simulink model "MLC_PreEval"  (Simulink 10.1)
settings: Solver=ode4  StartTime=0.0  StopTime=Parameter.Time.TMax  FixedStep=Parameter.Time.dt  MaxStep=10*Parameter.Time.dt  MinStep=Parameter.Time.dt  RelTol=1e-3  EnableMultiTasking=on
undefined symbols (not defined in the file or in its folder): Parameter, x2_t0
libraries: simulink x1
settings Model: Creator=Phoenix_Shao  LastModifiedBy=jveli
settings SolverCC: InitialStep=4*Parameter.Time.dt  MaxConsecutiveMinStep=10
settings DataIOCC: MaxDataPoints=1000000  SaveFormat=Dataset  SignalLogging=off  DSMLogging=off
settings OptimizationCC: ExpressionDepthLimit=2147483647  InitFltsAndDblsToZero=on  EfficientMapNaN2IntZero=off
settings DebuggingCC: SaveWithParameterizedLinksMsg=none  SignalResolutionControl=TryResolveAllWithWarning  SolverPrmCheckMsg=warning  MultiTaskDSMMsg=warning  MultiTaskCondExecSysMsg=none  FcnCallInpInsideContextMsg=warning  AllowSymbolicDim=off  StateNameClashWarn=warning
settings HardwareCC: TargetBitPerPointer=64  TargetBitPerSizeT=64  TargetBitPerPtrDiffT=64  TargetLongLongMode=on  TargetIntDivRoundTo=Zero  TargetEndianess=LittleEndian  TargetWordSize=64  TargetHWDeviceType=MATLAB Host  ProdEqTarget=off
settings ModelReferenceCC: ModelDependencies=|
  | MAP_x64.dll
  | OpenFAST-Simulink_x64.dll
  | FAST_SFunc.mexw64
settings SFSimCC: SimParseCustomCode=off
settings RTWCC: SystemTargetFile=accel.tlc  TemplateMakefile=accel_default_tmf  RTWVerbose=off
settings CodeAppCC: MaxIdLength=128
settings STFCustomTargetCC: MATLABClassNameForMDSCustomization=Simulink.SoftwareTarget.TargetSpecificTriggerConfigurationBase  SystemTargetFile=accel.tlc

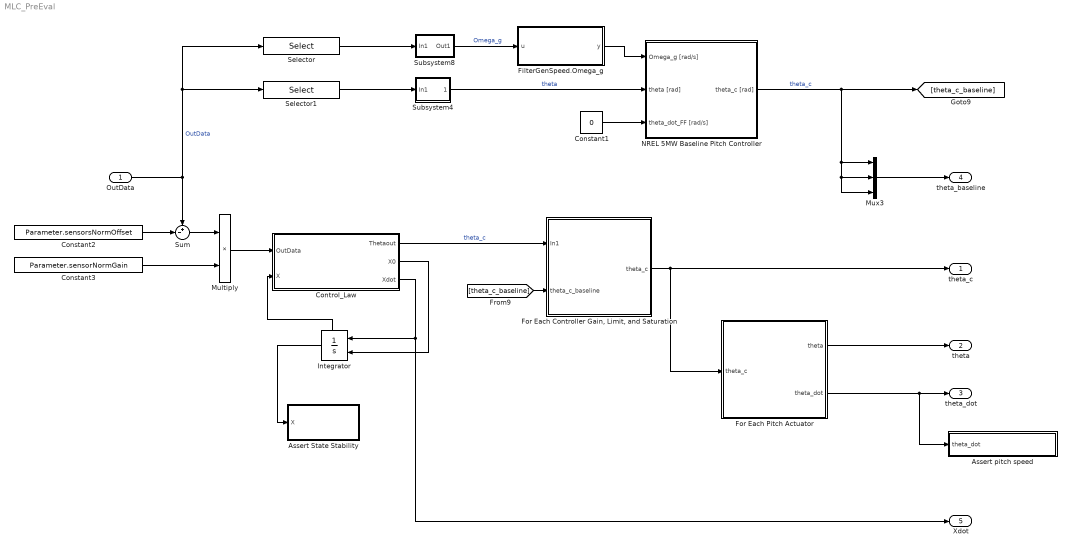
== system MLC_PreEval ==
  OutData : Inport  PortDimensions=Parameter.MLC.totNSensors
  Assert State Stability : Subsystem
  Assert pitch speed : Subsystem
  Constant1 : Constant  Value=0
  Constant2 : Constant  Value=Parameter.sensorsNormOffset
  Constant3 : Constant  Value=Parameter.sensorNormGain
  Control_Law : MATLAB Function  TreatAsAtomicUnit=on
  FilterGenSpeed.Omega_g : Subsystem
  For Each Pitch Actuator : Subsystem  TreatAsAtomicUnit=on
  "For Each Controller Gain, Limit, and Saturation" : Subsystem  TreatAsAtomicUnit=on
  Integrator : Integrator  InitialConditionSource=external  ShowStatePort=on
  Multiply : Product
  Mux3 : Mux  Inputs=3
  NREL 5MW Baseline Pitch Controller : Subsystem
  Selector : Selector  InputPortWidth=Parameter.outListLen  IndexOptions=Index vector (dialog)  Indices=Parameter.outListIdx.GenSpeed  OutputSizes=1
  Selector1 : Selector  InputPortWidth=Parameter.outListLen  IndexOptions=Index vector (dialog)  Indices=Parameter.outListIdx.BldPitch1  OutputSizes=1
  Subsystem4 : Subsystem
      mask Display: disp('deg2rad')
  Subsystem8 : Subsystem
      mask Display: disp('rpm2rad/s')
  Sum : Sum  Inputs=+-|
  "theta_c " : Outport  SignalName=theta_c  VectorParamsAs1DForOutWhenUnconnected=off
  theta : Outport  Port=2  SignalName=theta  VectorParamsAs1DForOutWhenUnconnected=off
  theta_dot : Outport  Port=3  SignalName=theta_dot  VectorParamsAs1DForOutWhenUnconnected=off
  theta_baseline : Outport  Port=4  SignalName=theta_baseline  VectorParamsAs1DForOutWhenUnconnected=off
  Xdot : Outport  Port=5  SignalName=Xdot  VectorParamsAs1DForOutWhenUnconnected=off
  wires:
  "For Each Controller Gain, Limit, and Saturation"/1(theta_c) -> For Each Pitch Actuator/1(theta_c), "theta_c "/1
  OutData/1 -> Selector1/1, Selector/1, Sum/1  "OutData"
  For Each Pitch Actuator/1(theta) -> theta/1
  For Each Pitch Actuator/2(theta_dot) -> Assert pitch speed/1(theta_dot), theta_dot/1
  FilterGenSpeed.Omega_g/1(y) -> NREL 5MW Baseline Pitch Controller/1(Omega_g [rad/s])
  Constant1/1 -> NREL 5MW Baseline Pitch Controller/3(theta_dot_FF [rad/s])
  Subsystem8/1(Out1) -> FilterGenSpeed.Omega_g/1(u)  "Omega_g"
  Selector/1 -> Subsystem8/1(In1)
  Subsystem4/1(Out1) -> NREL 5MW Baseline Pitch Controller/2(theta [rad])  "theta"
  Selector1/1 -> Subsystem4/1(In1)
  NREL 5MW Baseline Pitch Controller/1(theta_c [rad]) -> Mux3/1, Mux3/2, Mux3/3, [theta_c_baseline]  "theta_c"
  Constant2/1 -> Sum/2
  Sum/1 -> Multiply/1
  Constant3/1 -> Multiply/2
  Mux3/1 -> theta_baseline/1
  [theta_c_baseline] -> "For Each Controller Gain, Limit, and Saturation"/2(theta_c_baseline)
  Integrator/1 -> Assert State Stability/1(X)
  Control_Law/1(Thetaout) -> "For Each Controller Gain, Limit, and Saturation"/1(In1)  "theta_c"
  Control_Law/2(X0) -> Integrator/2
  Control_Law/3(Xdot) -> Xdot/1, Integrator/1
  Multiply/1 -> Control_Law/1(OutData)
  Integrator/State -> Control_Law/2(X)

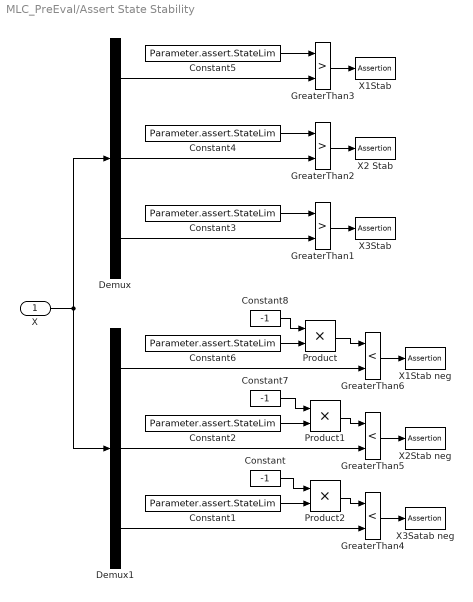
== system MLC_PreEval/Assert State Stability ==
  X : Inport
  Constant : Constant  Value=-1
  Constant{1..6} (6 alike) : Constant  Value=Parameter.assert.StateLim
  Constant7 : Constant  Value=-1
  Constant8 : Constant  Value=-1
  Demux : Demux  Outputs=3
  Demux1 : Demux  Outputs=3
  GreaterThan1 : RelationalOperator  Operator=>  OutDataTypeStr=boolean  RndMeth=Simplest
  GreaterThan2 : RelationalOperator  Operator=>  OutDataTypeStr=boolean  RndMeth=Simplest
  GreaterThan3 : RelationalOperator  Operator=>  OutDataTypeStr=boolean  RndMeth=Simplest
  GreaterThan4 : RelationalOperator  Operator=<  OutDataTypeStr=boolean  RndMeth=Simplest
  GreaterThan5 : RelationalOperator  Operator=<  OutDataTypeStr=boolean  RndMeth=Simplest
  GreaterThan6 : RelationalOperator  Operator=<  OutDataTypeStr=boolean  RndMeth=Simplest
  Product : Product
  Product1 : Product
  Product2 : Product
  X1Stab : Assertion
  X1Stab neg : Assertion
  X2 Stab : Assertion
  X2Stab neg : Assertion
  X3Satab neg : Assertion
  X3Stab : Assertion
  wires:
  Constant5/1 -> GreaterThan3/1
  GreaterThan1/1 -> X3Stab/1
  Constant3/1 -> GreaterThan1/1
  Constant4/1 -> GreaterThan2/1
  GreaterThan3/1 -> X1Stab/1
  GreaterThan2/1 -> X2 Stab/1
  X/1 -> Demux/1, Demux1/1
  Demux/2 -> GreaterThan2/2
  Demux/3 -> GreaterThan1/2
  GreaterThan6/1 -> X1Stab neg/1
  Demux/1 -> GreaterThan3/2
  GreaterThan4/1 -> X3Satab neg/1
  Constant2/1 -> Product1/2
  Constant6/1 -> Product/2
  Constant1/1 -> Product2/2
  GreaterThan5/1 -> X2Stab neg/1
  Product/1 -> GreaterThan6/1
  Product1/1 -> GreaterThan5/1
  Product2/1 -> GreaterThan4/1
  Constant/1 -> Product2/1
  Constant7/1 -> Product1/1
  Constant8/1 -> Product/1
  Demux1/2 -> GreaterThan5/2
  Demux1/1 -> GreaterThan6/2
  Demux1/3 -> GreaterThan4/2

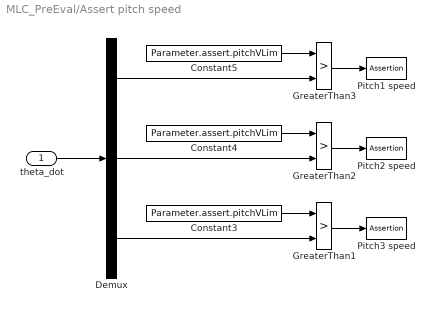
== system MLC_PreEval/Assert pitch speed ==
  theta_dot : Inport
  Constant3 : Constant  Value=Parameter.assert.pitchVLim
  Constant4 : Constant  Value=Parameter.assert.pitchVLim
  Constant5 : Constant  Value=Parameter.assert.pitchVLim
  Demux : Demux  Outputs=3
  GreaterThan1 : RelationalOperator  Operator=>  OutDataTypeStr=boolean  RndMeth=Simplest
  GreaterThan2 : RelationalOperator  Operator=>  OutDataTypeStr=boolean  RndMeth=Simplest
  GreaterThan3 : RelationalOperator  Operator=>  OutDataTypeStr=boolean  RndMeth=Simplest
  Pitch1 speed : Assertion
  Pitch2 speed : Assertion
  Pitch3 speed : Assertion
  wires:
  Constant5/1 -> GreaterThan3/1
  GreaterThan1/1 -> Pitch3 speed/1
  Constant3/1 -> GreaterThan1/1
  Constant4/1 -> GreaterThan2/1
  GreaterThan3/1 -> Pitch1 speed/1
  GreaterThan2/1 -> Pitch2 speed/1
  theta_dot/1 -> Demux/1
  Demux/1 -> GreaterThan3/2
  Demux/2 -> GreaterThan2/2
  Demux/3 -> GreaterThan1/2

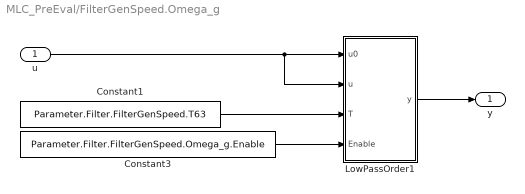
== system MLC_PreEval/FilterGenSpeed.Omega_g ==
  u : Inport
  Constant1 : Constant  Value=Parameter.Filter.FilterGenSpeed.T63
  Constant3 : Constant  Value=Parameter.Filter.FilterGenSpeed.Omega_g.Enable
  LowPassOrder1 : Subsystem
  y : Outport  VectorParamsAs1DForOutWhenUnconnected=off
  wires:
  LowPassOrder1/1(y) -> y/1
  u/1 -> LowPassOrder1/2(u), LowPassOrder1/1(u0)
  Constant3/1 -> LowPassOrder1/4(Enable)
  Constant1/1 -> LowPassOrder1/3(T)

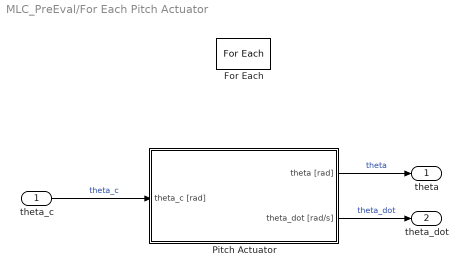
== system MLC_PreEval/For Each Pitch Actuator ==
  theta_c : Inport  Partition=on  PartitionDimension=1  PartitionWidth=1  PartitionOffset=0
  For Each : ForEach  DisableCoverage=on
  Pitch Actuator : Subsystem  AncestorBlock=Library/Models/Pitch Actuator
  theta : Outport  ConcatenationDimension=1  VectorParamsAs1DForOutWhenUnconnected=off
  theta_dot : Outport  Port=2  ConcatenationDimension=1  VectorParamsAs1DForOutWhenUnconnected=off
  wires:
  theta_c/1 -> Pitch Actuator/1(theta_c [rad])  "theta_c"
  Pitch Actuator/1(theta [rad]) -> theta/1  "theta"
  Pitch Actuator/2(theta_dot [rad/s]) -> theta_dot/1  "theta_dot"

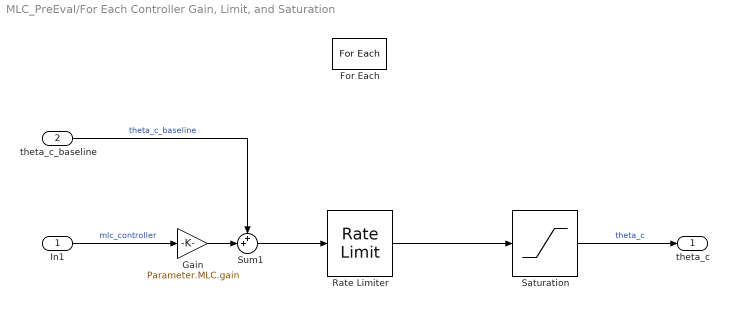
== system MLC_PreEval/For Each Controller Gain, Limit, and Saturation ==
  In1 : Inport  Partition=on  PartitionDimension=1  PartitionWidth=1  PartitionOffset=0
  theta_c_baseline : Inport  Port=2
  For Each : ForEach  DisableCoverage=on
  Gain : Gain  Gain=Parameter.MLC.gain
      settings: AttributesFormatString=%<Gain>
  Rate Limiter : RateLimiter  RisingSlewLimit=deg2rad(Parameter.assert.pitchVLim)  FallingSlewLimit=-deg2rad(Parameter.assert.pitchVLim)  SampleTimeMode=inherited
      settings: AttributesFormatString=|
      | %<RisingSlewLimit>
      | %<FallingSlewLimit>
  Saturation : Saturate  UpperLimit=Parameter.CPC.theta_max  LowerLimit=Parameter.CPC.theta_min
      settings: AttributesFormatString=|
      | %<UpperLimit>
      | %<LowerLimit>
  Sum1 : Sum  Inputs=++|
  theta_c : Outport  ConcatenationDimension=1  VectorParamsAs1DForOutWhenUnconnected=off
  wires:
  Sum1/1 -> Rate Limiter/1
  Saturation/1 -> theta_c/1  "theta_c"
  Gain/1 -> Sum1/2
  theta_c_baseline/1 -> Sum1/1  "theta_c_baseline"
  Rate Limiter/1 -> Saturation/1
  In1/1 -> Gain/1  "mlc_controller"

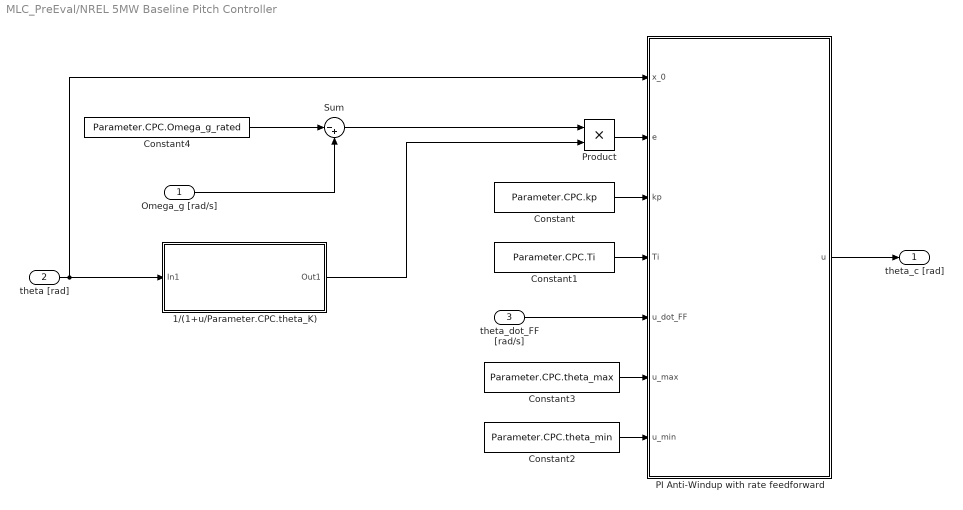
== system MLC_PreEval/NREL 5MW Baseline Pitch Controller ==
  Omega_g [rad/s] : Inport
  theta [rad] : Inport  Port=2
  theta_dot_FF [rad/s] : Inport  Port=3
  1/(1+u/Parameter.CPC.theta_K) : Subsystem
  Constant : Constant  Value=Parameter.CPC.kp
  Constant1 : Constant  Value=Parameter.CPC.Ti
  Constant2 : Constant  Value=Parameter.CPC.theta_min
  Constant3 : Constant  Value=Parameter.CPC.theta_max
  Constant4 : Constant  Value=Parameter.CPC.Omega_g_rated
  PI Anti-Windup with rate feedforward : Subsystem
  Product : Product  RndMeth=Zero
  Sum : Sum  Inputs=|-+
  theta_c [rad] : Outport  VectorParamsAs1DForOutWhenUnconnected=off
  wires:
  Constant4/1 -> Sum/1
  theta [rad]/1 -> 1/(1+u/Parameter.CPC.theta_K)/1(In1), PI Anti-Windup with rate feedforward/1(x_0)
  Omega_g [rad/s]/1 -> Sum/2
  1/(1+u/Parameter.CPC.theta_K)/1(Out1) -> Product/2
  Sum/1 -> Product/1
  Product/1 -> PI Anti-Windup with rate feedforward/2(e)
  theta_dot_FF [rad/s]/1 -> PI Anti-Windup with rate feedforward/5(u_dot_FF)
  PI Anti-Windup with rate feedforward/1(u) -> theta_c [rad]/1
  Constant/1 -> PI Anti-Windup with rate feedforward/3(kp)
  Constant1/1 -> PI Anti-Windup with rate feedforward/4(Ti)
  Constant2/1 -> PI Anti-Windup with rate feedforward/7(u_min)
  Constant3/1 -> PI Anti-Windup with rate feedforward/6(u_max)

== system MLC_PreEval/Subsystem4 ==
  In1 : Inport
  deg in rad : Gain  Gain=2*pi/360  SaturateOnIntegerOverflow=on  OutDataTypeStr=Inherit: Same as input  ParamDataTypeStr=Inherit: Same as input
  Out1 : Outport  VectorParamsAs1DForOutWhenUnconnected=off
  wires:
  In1/1 -> deg in rad/1
  deg in rad/1 -> Out1/1

== system MLC_PreEval/Subsystem8 ==
  In1 : Inport
  rpm in rad/s : Gain  Gain=2*pi/60  SaturateOnIntegerOverflow=on  OutDataTypeStr=Inherit: Same as input  ParamDataTypeStr=Inherit: Same as input
  Out1 : Outport  VectorParamsAs1DForOutWhenUnconnected=off
  wires:
  rpm in rad/s/1 -> Out1/1
  In1/1 -> rpm in rad/s/1

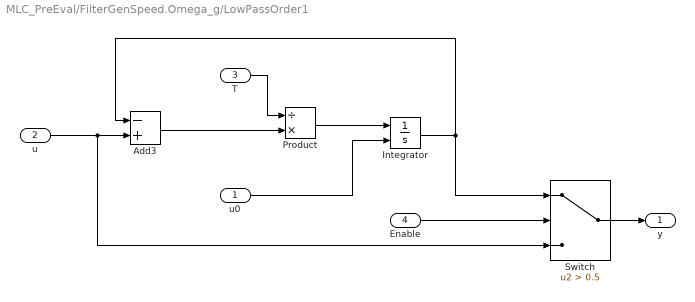
== system MLC_PreEval/FilterGenSpeed.Omega_g/LowPassOrder1 ==
  u0 : Inport
  u : Inport  Port=2
  T : Inport  Port=3
  Enable : Inport  Port=4
  Add3 : Sum  Inputs=-+
  Integrator : Integrator  InitialConditionSource=external
  Product : Product  Inputs=/*  RndMeth=Zero
  Switch : Switch  Criteria=u2 > Threshold  Threshold=0.5
  y : Outport  VectorParamsAs1DForOutWhenUnconnected=off
  wires:
  u0/1 -> Integrator/2
  Switch/1 -> y/1
  Enable/1 -> Switch/2
  u/1 -> Add3/2, Switch/3
  T/1 -> Product/1
  Integrator/1 -> Add3/1, Switch/1
  Product/1 -> Integrator/1
  Add3/1 -> Product/2

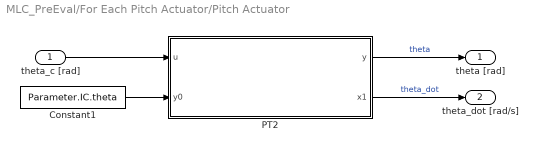
== system MLC_PreEval/For Each Pitch Actuator/Pitch Actuator ==
  theta_c [rad] : Inport
  Constant1 : Constant  Value=Parameter.IC.theta
  PT2 : Subsystem  mask{omega=Parameter.PitchActuator.omega, xi=Parameter.PitchActuator.xi, x1_max=Parameter.PitchActuator.theta_dot_max, x1_min=-Parameter.PitchActuator.theta_dot_max, x2_max=Parameter.PitchActuator.theta_max, x2_min=Parameter.PitchActuator.theta_min}
      mask prompts: omega "undamped natural frequency [rad/s]"; xi "damping factor [-]"; x1_max "Upper bound x1"; x1_min "Lower bound x1"; x2_max "Upper bound x2"; x2_min "Lower bound x2"
      mask Display:
      | disp(['omega = ',num2str(omega),'\n'...
      |     ,'xi = ',num2str(xi)])
      | port_label('output',1,'y')
      | port_label('output',2,'x1')
      | port_label('input',2,'y0')
      | port_label('input',1,'u')
  theta [rad] : Outport  VectorParamsAs1DForOutWhenUnconnected=off
  theta_dot [rad/s] : Outport  Port=2  VectorParamsAs1DForOutWhenUnconnected=off
  wires:
  Constant1/1 -> PT2/2(y0)
  theta_c [rad]/1 -> PT2/1(u)
  PT2/1(y) -> theta [rad]/1  "theta"
  PT2/2(x1) -> theta_dot [rad/s]/1  "theta_dot"

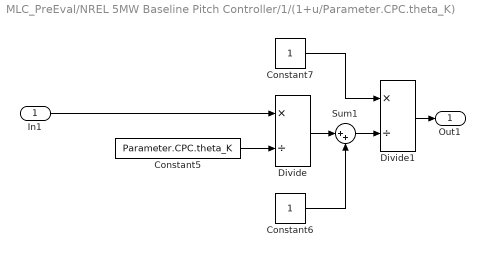
== system MLC_PreEval/NREL 5MW Baseline Pitch Controller/1/(1+u/Parameter.CPC.theta_K) ==
  In1 : Inport
  Constant5 : Constant  Value=Parameter.CPC.theta_K
  Constant6 : Constant
  Constant7 : Constant
  Divide : Product  Inputs=*/
  Divide1 : Product  Inputs=*/
  Sum1 : Sum  Inputs=|++
  Out1 : Outport  VectorParamsAs1DForOutWhenUnconnected=off
  wires:
  Sum1/1 -> Divide1/2
  Divide/1 -> Sum1/1
  In1/1 -> Divide/1
  Divide1/1 -> Out1/1
  Constant7/1 -> Divide1/1
  Constant5/1 -> Divide/2
  Constant6/1 -> Sum1/2

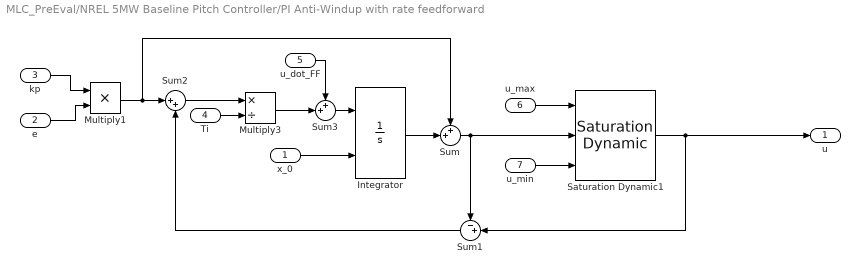
== system MLC_PreEval/NREL 5MW Baseline Pitch Controller/PI Anti-Windup with rate feedforward ==
  x_0 : Inport
  e : Inport  Port=2
  kp : Inport  Port=3
  Ti : Inport  Port=4
  u_dot_FF : Inport  Port=5
  u_max : Inport  Port=6
  u_min : Inport  Port=7
  Integrator : Integrator  InitialConditionSource=external
  Multiply1 : Product  Inputs=**
  Multiply3 : Product  Inputs=*/
  Saturation Dynamic1 : simulink/Discontinuities/Saturation Dynamic  OutMin=[]  OutMax=[]  OutDataTypeStr=Inherit: Same as second input  OutDataType=fixdt(1, 16)  OutScaling=2^-10  DoSatur=off
  Sum : Sum  Inputs=++|
  Sum1 : Sum  Inputs=-+|
  Sum2 : Sum  Inputs=|++
  Sum3 : Sum  Inputs=++|
  u : Outport  VectorParamsAs1DForOutWhenUnconnected=off
  wires:
  Saturation Dynamic1/1 -> u/1, Sum1/2
  Integrator/1 -> Sum/2
  kp/1 -> Multiply1/1
  e/1 -> Multiply1/2
  Ti/1 -> Multiply3/2
  Multiply1/1 -> Sum/1, Sum2/1
  Sum2/1 -> Multiply3/1
  x_0/1 -> Integrator/2
  Multiply3/1 -> Sum3/2
  Sum3/1 -> Integrator/1
  u_dot_FF/1 -> Sum3/1
  u_min/1 -> Saturation Dynamic1/3
  Sum/1 -> Saturation Dynamic1/2, Sum1/1
  u_max/1 -> Saturation Dynamic1/1
  Sum1/1 -> Sum2/2

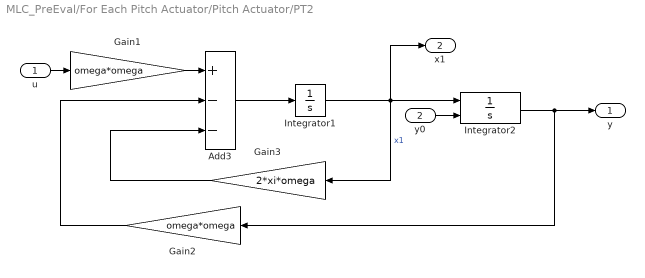
== system MLC_PreEval/For Each Pitch Actuator/Pitch Actuator/PT2 ==
  u : Inport
  y0 : Inport  Port=2
  Add3 : Sum  Inputs=+--
  Gain1 : Gain  Gain=omega*omega  SaturateOnIntegerOverflow=on  OutDataTypeStr=Inherit: Same as input  ParamDataTypeStr=Inherit: Same as input
  Gain2 : Gain  Gain=omega*omega  SaturateOnIntegerOverflow=on  OutDataTypeStr=Inherit: Same as input  ParamDataTypeStr=Inherit: Same as input
  Gain3 : Gain  Gain=2*xi*omega  SaturateOnIntegerOverflow=on  OutDataTypeStr=Inherit: Same as input  ParamDataTypeStr=Inherit: Same as input
  Integrator1 : Integrator  LimitOutput=on  UpperSaturationLimit=x1_max  LowerSaturationLimit=x1_min
  Integrator2 : Integrator  InitialConditionSource=external  InitialCondition=x2_t0  LimitOutput=on  UpperSaturationLimit=x2_max  LowerSaturationLimit=x2_min
  y : Outport  VectorParamsAs1DForOutWhenUnconnected=off
  x1 : Outport  Port=2  VectorParamsAs1DForOutWhenUnconnected=off
  wires:
  Integrator2/1 -> y/1, Gain2/1
  y0/1 -> Integrator2/2
  Integrator1/1 -> Integrator2/1, Gain3/1, x1/1  "x1"
  Gain2/1 -> Add3/2
  Gain1/1 -> Add3/1
  Add3/1 -> Integrator1/1
  u/1 -> Gain1/1
  Gain3/1 -> Add3/3

== matlab function Control_Law ==
  data: Thetaout output double; X0 output double; Xdot output double; OutData input double; X input double; CParameter parameter double
function [Thetaout, X0, Xdot] = ControlLaw(OutData, X, CParameter)

Thetaout = [1; 1; 1];
X0 = [0; 0];
Xdot = [0; 0];

end
